simulink model "visualisation_system"  (R2014a)
settings: Solver=VariableStepDiscrete  StartTime=0.0  StopTime=36e4  FixedStep=60  MaxStep=300  RelTol=1e-3
libraries: vrlib x3
settings Model: Creator=Piotr  LastModifiedBy=Piotr
settings OptimizationCC: SimCompilerOptimization=off
settings DebuggingCC: UnderspecifiedInitializationDetection=Classic  FrameProcessingCompatibilityMsg=error  StateNameClashWarn=warning
settings RTWCC: RTWCompilerOptimization=off

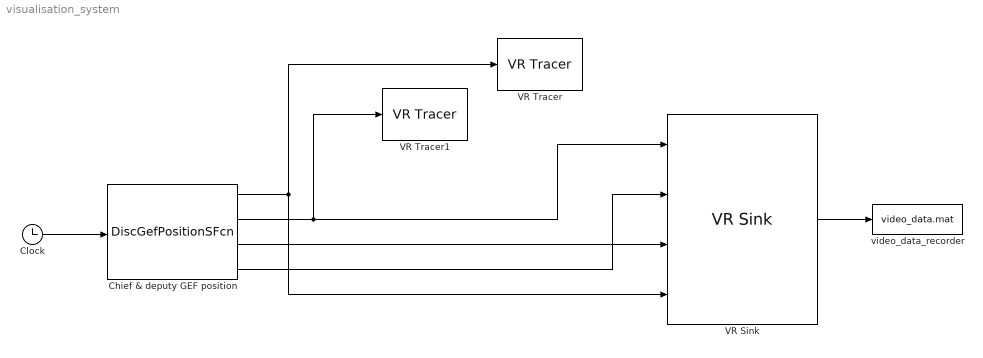
== system visualisation_system ==
  Chief & deputy GEF position : M-S-Function  FunctionName=DiscGefPositionSFcn  Parameters=ResAnalysis
  Clock : Clock
  VR Sink : vrlib/VR Sink  InstantiateOnLoad=on  SampleTime=-1  ViewEnable=on  RemoteChange=off  RemoteView=off  FieldsWritten=Deputy.translation#DeputyInitPos.translation#ChiefInitPos.translation#Chief.translation  WorldFileName=orbits.wrl  AutoView=off  VideoDimensions=[640 960]  AllowVariableSize=off  FigureProperties="{'Position', 'Name', 'Viewpoint', 'CameraBound', 'CameraDirection', 'CameraPosition', 'CameraUpVector', 'ZoomFactor', 'Antialiasing', 'Headlight', 'Lighting', 'NavPanel', 'StatusBar', 'ToolBar', 'Textures', 'Transparency', 'Triad', 'Wireframe', 'NavZones', 'NavMode', 'NavSpeed', 'CaptureFileFormat', 'CaptureFileName', 'Record2DCompressMethod', 'Record2DCompressQuality', 'Record2D', 'Record2DFileName', 'Record2DFPS'; [3.0000000000000000e+01   6.0000000000000000e+01   9.6000000000000000e+02   6.4000000000000000e+02], '', 'VP1', 'on', [-6.4734291958420109e-01   4.7322926888582673e-01   5.9749577700096457e-01], [4.0460371549199230e+01  -3.1712177100633028e+01  -9.8968398407557629e+01], [2.8029932982030398e-01  -5.8117174550928841e-01   7.6398408878979607e-01], [1.0000000000000000e+00], 'on', 'on', 'on', 'none', 'off', 'off', 'on', 'on', 'none', 'off', 'off', 'examine', 'normal', 'tif', '%f_anim_%n.tif', 'auto', [7.5000000000000000e+01], 'off', '***video***', 'auto'}"
  VR Tracer : vrlib/VR Tracer  VrmlFile=orbits.wrl  MarkerName=None  UseLines=on  UseTriads=off  MarkerScale=[1 1 1]  MarkerColorSelection=Defined as RGB values  MarkerColor=red  rgbval=[0.5 0 0]  ConnectPlane=off  PlaneCoeff=[0 1 0 0]  ConnectPoint=None  PointCoord=[0 0 0]  Ts=-1  ForceViewerOpen=off
  VR Tracer1 : vrlib/VR Tracer  VrmlFile=orbits.wrl  MarkerName=None  UseLines=on  UseTriads=off  MarkerScale=[1 1 1]  MarkerColorSelection=Defined as RGB values  MarkerColor=red  rgbval=[0 0.5 0]  ConnectPlane=off  PlaneCoeff=[0 1 0 0]  ConnectPoint=None  PointCoord=[0 0 0]  Ts=-1  ForceViewerOpen=off
  video_data_recorder : ToFile  Filename=video_data.mat  MatrixName=video_data  SaveFormat=Timeseries  SampleTime=1200
      settings: AttributesFormatString=%<SampleTime>
  wires:
  Chief & deputy GEF position/2 -> VR Sink/1, VR Tracer1/1
  Clock/1 -> Chief & deputy GEF position/1
  VR Sink/1 -> video_data_recorder/1
  Chief & deputy GEF position/1 -> VR Sink/4, VR Tracer/1
  Chief & deputy GEF position/4 -> VR Sink/2
  Chief & deputy GEF position/3 -> VR Sink/3
